simulink model "DataPath"  (R2025a)
settings: Solver=FixedStepAuto  StartTime=0  StopTime=0.02  FixedStep=1e-7  RelTol=1e-3
undefined symbols (not defined in the file): Bit_1, Bit_2, Bit_3, Bit_4, Bit_5, Bit_6, Bit_7, Bit_8
libraries: simulink_extras x126, fl_lib x34, nesl_utility x18, simulink x2
(part 7 of 7)

== system DataPath/Subsystem1/ALU Regs/B2/Subsystem4 ==
  Data : Inport
  Store : Inport  Port=2
  Clock : Inport  Port=3
  Clear : Inport  Port=4
  AND : Logic  IconShape=distinctive  AllPortsSameDT=off  OutDataTypeStr=boolean
  AND1 : Logic  IconShape=distinctive  AllPortsSameDT=off  OutDataTypeStr=boolean
  D Flip-Flop : simulink_extras/Flip Flops/D Flip-Flop
  NOT : Logic  Operator=NOT  IconShape=distinctive  AllPortsSameDT=off  OutDataTypeStr=boolean
  NOT1 : Logic  Operator=NOT  IconShape=distinctive  AllPortsSameDT=off  OutDataTypeStr=boolean
  OR : Logic  Operator=OR  IconShape=distinctive  AllPortsSameDT=off  OutDataTypeStr=boolean
  Q : Outport
  !Q : Outport  Port=2
  wires:
  AND1/1 -> OR/2
  AND/1 -> OR/1
  D Flip-Flop/1 -> Q/1, AND1/2
  NOT/1 -> AND1/1
  Store/1 -> AND/2, NOT/1
  Clock/1 -> D Flip-Flop/2
  Data/1 -> AND/1
  OR/1 -> D Flip-Flop/1
  D Flip-Flop/2 -> !Q/1
  Clear/1 -> NOT1/1
  NOT1/1 -> D Flip-Flop/3

== system DataPath/Subsystem1/ALU Regs/B2/Subsystem5 ==
  Data : Inport
  Store : Inport  Port=2
  Clock : Inport  Port=3
  Clear : Inport  Port=4
  AND : Logic  IconShape=distinctive  AllPortsSameDT=off  OutDataTypeStr=boolean
  AND1 : Logic  IconShape=distinctive  AllPortsSameDT=off  OutDataTypeStr=boolean
  D Flip-Flop : simulink_extras/Flip Flops/D Flip-Flop
  NOT : Logic  Operator=NOT  IconShape=distinctive  AllPortsSameDT=off  OutDataTypeStr=boolean
  NOT1 : Logic  Operator=NOT  IconShape=distinctive  AllPortsSameDT=off  OutDataTypeStr=boolean
  OR : Logic  Operator=OR  IconShape=distinctive  AllPortsSameDT=off  OutDataTypeStr=boolean
  Q : Outport
  !Q : Outport  Port=2
  wires:
  AND1/1 -> OR/2
  AND/1 -> OR/1
  D Flip-Flop/1 -> Q/1, AND1/2
  NOT/1 -> AND1/1
  Store/1 -> AND/2, NOT/1
  Clock/1 -> D Flip-Flop/2
  Data/1 -> AND/1
  OR/1 -> D Flip-Flop/1
  D Flip-Flop/2 -> !Q/1
  Clear/1 -> NOT1/1
  NOT1/1 -> D Flip-Flop/3

== system DataPath/Subsystem1/ALU Regs/B2/Subsystem6 ==
  Data : Inport
  Store : Inport  Port=2
  Clock : Inport  Port=3
  Clear : Inport  Port=4
  AND : Logic  IconShape=distinctive  AllPortsSameDT=off  OutDataTypeStr=boolean
  AND1 : Logic  IconShape=distinctive  AllPortsSameDT=off  OutDataTypeStr=boolean
  D Flip-Flop : simulink_extras/Flip Flops/D Flip-Flop
  NOT : Logic  Operator=NOT  IconShape=distinctive  AllPortsSameDT=off  OutDataTypeStr=boolean
  NOT1 : Logic  Operator=NOT  IconShape=distinctive  AllPortsSameDT=off  OutDataTypeStr=boolean
  OR : Logic  Operator=OR  IconShape=distinctive  AllPortsSameDT=off  OutDataTypeStr=boolean
  Q : Outport
  !Q : Outport  Port=2
  wires:
  AND1/1 -> OR/2
  AND/1 -> OR/1
  D Flip-Flop/1 -> Q/1, AND1/2
  NOT/1 -> AND1/1
  Store/1 -> AND/2, NOT/1
  Clock/1 -> D Flip-Flop/2
  Data/1 -> AND/1
  OR/1 -> D Flip-Flop/1
  D Flip-Flop/2 -> !Q/1
  Clear/1 -> NOT1/1
  NOT1/1 -> D Flip-Flop/3

== system DataPath/Subsystem1/ALU Regs/B2/Subsystem7 ==
  Data : Inport
  Store : Inport  Port=2
  Clock : Inport  Port=3
  Clear : Inport  Port=4
  AND : Logic  IconShape=distinctive  AllPortsSameDT=off  OutDataTypeStr=boolean
  AND1 : Logic  IconShape=distinctive  AllPortsSameDT=off  OutDataTypeStr=boolean
  D Flip-Flop : simulink_extras/Flip Flops/D Flip-Flop
  NOT : Logic  Operator=NOT  IconShape=distinctive  AllPortsSameDT=off  OutDataTypeStr=boolean
  NOT1 : Logic  Operator=NOT  IconShape=distinctive  AllPortsSameDT=off  OutDataTypeStr=boolean
  OR : Logic  Operator=OR  IconShape=distinctive  AllPortsSameDT=off  OutDataTypeStr=boolean
  Q : Outport
  !Q : Outport  Port=2
  wires:
  AND1/1 -> OR/2
  AND/1 -> OR/1
  D Flip-Flop/1 -> Q/1, AND1/2
  NOT/1 -> AND1/1
  Store/1 -> AND/2, NOT/1
  Clock/1 -> D Flip-Flop/2
  Data/1 -> AND/1
  OR/1 -> D Flip-Flop/1
  D Flip-Flop/2 -> !Q/1
  Clear/1 -> NOT1/1
  NOT1/1 -> D Flip-Flop/3

== system DataPath/Subsystem1/ALU Regs/B2/Subsystem8 ==
  Data : Inport
  Store : Inport  Port=2
  Clock : Inport  Port=3
  Clear : Inport  Port=4
  AND : Logic  IconShape=distinctive  AllPortsSameDT=off  OutDataTypeStr=boolean
  AND1 : Logic  IconShape=distinctive  AllPortsSameDT=off  OutDataTypeStr=boolean
  D Flip-Flop : simulink_extras/Flip Flops/D Flip-Flop
  NOT : Logic  Operator=NOT  IconShape=distinctive  AllPortsSameDT=off  OutDataTypeStr=boolean
  NOT1 : Logic  Operator=NOT  IconShape=distinctive  AllPortsSameDT=off  OutDataTypeStr=boolean
  OR : Logic  Operator=OR  IconShape=distinctive  AllPortsSameDT=off  OutDataTypeStr=boolean
  Q : Outport
  !Q : Outport  Port=2
  wires:
  AND1/1 -> OR/2
  AND/1 -> OR/1
  D Flip-Flop/1 -> Q/1, AND1/2
  NOT/1 -> AND1/1
  Store/1 -> AND/2, NOT/1
  Clock/1 -> D Flip-Flop/2
  Data/1 -> AND/1
  OR/1 -> D Flip-Flop/1
  D Flip-Flop/2 -> !Q/1
  Clear/1 -> NOT1/1
  NOT1/1 -> D Flip-Flop/3

== system DataPath/Subsystem1/Normalize Div/Subsystem1/Subsystem6 ==
  Data : Inport
  CLK : Inport  Port=2
  Delay One Step : Delay  DelayLength=1
  NAND{1..4} (4 alike) : Logic  Operator=NAND  IconShape=distinctive  AllPortsSameDT=off  OutDataTypeStr=boolean
  Q : Outport
  !Q : Outport  Port=2
  wires:
  NAND1/1 -> Delay One Step/1
  NAND4/1 -> NAND2/2
  Delay One Step/1 -> NAND2/1, Q/1  "Q"
  NAND2/1 -> !Q/1, NAND1/2
  NAND3/1 -> NAND4/1, NAND1/1
  CLK/1 -> NAND3/2, NAND4/2
  Data/1 -> NAND3/1

== system DataPath/Subsystem1/Normalize Div/Subsystem1/Subsystem7 ==
  Data : Inport
  CLK : Inport  Port=2
  Delay One Step : Delay  DelayLength=1
  NAND{1..4} (4 alike) : Logic  Operator=NAND  IconShape=distinctive  AllPortsSameDT=off  OutDataTypeStr=boolean
  Q : Outport
  !Q : Outport  Port=2
  wires:
  NAND1/1 -> Delay One Step/1
  NAND4/1 -> NAND2/2
  Delay One Step/1 -> NAND2/1, Q/1  "Q"
  NAND2/1 -> !Q/1, NAND1/2
  NAND3/1 -> NAND4/1, NAND1/1
  CLK/1 -> NAND3/2, NAND4/2
  Data/1 -> NAND3/1

== system DataPath/Subsystem1/Normalize Div/Subsystem8/Subsystem6 ==
  Data : Inport
  CLK : Inport  Port=2
  Delay One Step : Delay  DelayLength=1
  NAND{1..4} (4 alike) : Logic  Operator=NAND  IconShape=distinctive  AllPortsSameDT=off  OutDataTypeStr=boolean
  Q : Outport
  !Q : Outport  Port=2
  wires:
  NAND1/1 -> Delay One Step/1
  NAND4/1 -> NAND2/2
  Delay One Step/1 -> NAND2/1, Q/1  "Q"
  NAND2/1 -> !Q/1, NAND1/2
  NAND3/1 -> NAND4/1, NAND1/1
  CLK/1 -> NAND3/2, NAND4/2
  Data/1 -> NAND3/1

== system DataPath/Subsystem1/Normalize Div/Subsystem8/Subsystem7 ==
  Data : Inport
  CLK : Inport  Port=2
  Delay One Step : Delay  DelayLength=1
  NAND{1..4} (4 alike) : Logic  Operator=NAND  IconShape=distinctive  AllPortsSameDT=off  OutDataTypeStr=boolean
  Q : Outport
  !Q : Outport  Port=2
  wires:
  NAND1/1 -> Delay One Step/1
  NAND4/1 -> NAND2/2
  Delay One Step/1 -> NAND2/1, Q/1  "Q"
  NAND2/1 -> !Q/1, NAND1/2
  NAND3/1 -> NAND4/1, NAND1/1
  CLK/1 -> NAND3/2, NAND4/2
  Data/1 -> NAND3/1

== system DataPath/Subsystem1/Stepper/Subsystem1/DFF ==
  Data : Inport
  CLK : Inport  Port=2
  DLatch Master : Subsystem
  DLatch Slave : Subsystem
  NOT6 : Logic  Operator=NOT  IconShape=distinctive  AllPortsSameDT=off  OutDataTypeStr=boolean
  Q : Outport
  !Q : Outport  Port=2
  wires:
  DLatch Master/1(Q) -> DLatch Slave/1(Data)
  NOT6/1 -> DLatch Master/2(CLK)
  CLK/1 -> DLatch Slave/2(CLK), NOT6/1
  Data/1 -> DLatch Master/1(Data)
  DLatch Slave/1(Q) -> Q/1
  DLatch Slave/2(!Q) -> !Q/1

== system DataPath/Subsystem1/Stepper/Subsystem2/DFF ==
  Data : Inport
  CLK : Inport  Port=2
  DLatch Master : Subsystem
  DLatch Slave : Subsystem
  NOT6 : Logic  Operator=NOT  IconShape=distinctive  AllPortsSameDT=off  OutDataTypeStr=boolean
  Q : Outport
  !Q : Outport  Port=2
  wires:
  DLatch Master/1(Q) -> DLatch Slave/1(Data)
  NOT6/1 -> DLatch Master/2(CLK)
  CLK/1 -> DLatch Slave/2(CLK), NOT6/1
  Data/1 -> DLatch Master/1(Data)
  DLatch Slave/1(Q) -> Q/1
  DLatch Slave/2(!Q) -> !Q/1

== system DataPath/Subsystem1/Stepper/Subsystem3/DFF ==
  Data : Inport
  CLK : Inport  Port=2
  DLatch Master : Subsystem
  DLatch Slave : Subsystem
  NOT6 : Logic  Operator=NOT  IconShape=distinctive  AllPortsSameDT=off  OutDataTypeStr=boolean
  Q : Outport
  !Q : Outport  Port=2
  wires:
  DLatch Master/1(Q) -> DLatch Slave/1(Data)
  NOT6/1 -> DLatch Master/2(CLK)
  CLK/1 -> DLatch Slave/2(CLK), NOT6/1
  Data/1 -> DLatch Master/1(Data)
  DLatch Slave/1(Q) -> Q/1
  DLatch Slave/2(!Q) -> !Q/1

== system DataPath/Subsystem1/Stepper/Subsystem4/DFF ==
  Data : Inport
  CLK : Inport  Port=2
  DLatch Master : Subsystem
  DLatch Slave : Subsystem
  NOT6 : Logic  Operator=NOT  IconShape=distinctive  AllPortsSameDT=off  OutDataTypeStr=boolean
  Q : Outport
  !Q : Outport  Port=2
  wires:
  DLatch Master/1(Q) -> DLatch Slave/1(Data)
  NOT6/1 -> DLatch Master/2(CLK)
  CLK/1 -> DLatch Slave/2(CLK), NOT6/1
  Data/1 -> DLatch Master/1(Data)
  DLatch Slave/1(Q) -> Q/1
  DLatch Slave/2(!Q) -> !Q/1

== system DataPath/Subsystem/Stepper/Subsystem1/DFF/DLatch Master ==
  Data : Inport
  CLK : Inport  Port=2
  Delay One Step : Delay  DelayLength=1
  NAND{1..4} (4 alike) : Logic  Operator=NAND  IconShape=distinctive  AllPortsSameDT=off  OutDataTypeStr=boolean
  Q : Outport
  !Q : Outport  Port=2
  wires:
  NAND1/1 -> Delay One Step/1
  NAND4/1 -> NAND2/2
  Delay One Step/1 -> NAND2/1, Q/1  "Q"
  NAND2/1 -> !Q/1, NAND1/2
  NAND3/1 -> NAND4/1, NAND1/1
  CLK/1 -> NAND3/2, NAND4/2
  Data/1 -> NAND3/1

== system DataPath/Subsystem/Stepper/Subsystem1/DFF/DLatch Slave ==
  Data : Inport
  CLK : Inport  Port=2
  Delay One Step : Delay  DelayLength=1
  NAND{1..4} (4 alike) : Logic  Operator=NAND  IconShape=distinctive  AllPortsSameDT=off  OutDataTypeStr=boolean
  Q : Outport
  !Q : Outport  Port=2
  wires:
  NAND1/1 -> Delay One Step/1
  NAND4/1 -> NAND2/2
  Delay One Step/1 -> NAND2/1, Q/1  "Q"
  NAND2/1 -> !Q/1, NAND1/2
  NAND3/1 -> NAND4/1, NAND1/1
  CLK/1 -> NAND3/2, NAND4/2
  Data/1 -> NAND3/1

== system DataPath/Subsystem/Stepper/Subsystem2/DFF/DLatch Master ==
  Data : Inport
  CLK : Inport  Port=2
  Delay One Step : Delay  DelayLength=1
  NAND{1..4} (4 alike) : Logic  Operator=NAND  IconShape=distinctive  AllPortsSameDT=off  OutDataTypeStr=boolean
  Q : Outport
  !Q : Outport  Port=2
  wires:
  NAND1/1 -> Delay One Step/1
  NAND4/1 -> NAND2/2
  Delay One Step/1 -> NAND2/1, Q/1  "Q"
  NAND2/1 -> !Q/1, NAND1/2
  NAND3/1 -> NAND4/1, NAND1/1
  CLK/1 -> NAND3/2, NAND4/2
  Data/1 -> NAND3/1

== system DataPath/Subsystem/Stepper/Subsystem2/DFF/DLatch Slave ==
  Data : Inport
  CLK : Inport  Port=2
  Delay One Step : Delay  DelayLength=1
  NAND{1..4} (4 alike) : Logic  Operator=NAND  IconShape=distinctive  AllPortsSameDT=off  OutDataTypeStr=boolean
  Q : Outport
  !Q : Outport  Port=2
  wires:
  NAND1/1 -> Delay One Step/1
  NAND4/1 -> NAND2/2
  Delay One Step/1 -> NAND2/1, Q/1  "Q"
  NAND2/1 -> !Q/1, NAND1/2
  NAND3/1 -> NAND4/1, NAND1/1
  CLK/1 -> NAND3/2, NAND4/2
  Data/1 -> NAND3/1

== system DataPath/Subsystem/Stepper/Subsystem3/DFF/DLatch Master ==
  Data : Inport
  CLK : Inport  Port=2
  Delay One Step : Delay  DelayLength=1
  NAND{1..4} (4 alike) : Logic  Operator=NAND  IconShape=distinctive  AllPortsSameDT=off  OutDataTypeStr=boolean
  Q : Outport
  !Q : Outport  Port=2
  wires:
  NAND1/1 -> Delay One Step/1
  NAND4/1 -> NAND2/2
  Delay One Step/1 -> NAND2/1, Q/1  "Q"
  NAND2/1 -> !Q/1, NAND1/2
  NAND3/1 -> NAND4/1, NAND1/1
  CLK/1 -> NAND3/2, NAND4/2
  Data/1 -> NAND3/1

== system DataPath/Subsystem/Stepper/Subsystem3/DFF/DLatch Slave ==
  Data : Inport
  CLK : Inport  Port=2
  Delay One Step : Delay  DelayLength=1
  NAND{1..4} (4 alike) : Logic  Operator=NAND  IconShape=distinctive  AllPortsSameDT=off  OutDataTypeStr=boolean
  Q : Outport
  !Q : Outport  Port=2
  wires:
  NAND1/1 -> Delay One Step/1
  NAND4/1 -> NAND2/2
  Delay One Step/1 -> NAND2/1, Q/1  "Q"
  NAND2/1 -> !Q/1, NAND1/2
  NAND3/1 -> NAND4/1, NAND1/1
  CLK/1 -> NAND3/2, NAND4/2
  Data/1 -> NAND3/1

== system DataPath/Subsystem/Stepper/Subsystem4/DFF/DLatch Master ==
  Data : Inport
  CLK : Inport  Port=2
  Delay One Step : Delay  DelayLength=1
  NAND{1..4} (4 alike) : Logic  Operator=NAND  IconShape=distinctive  AllPortsSameDT=off  OutDataTypeStr=boolean
  Q : Outport
  !Q : Outport  Port=2
  wires:
  NAND1/1 -> Delay One Step/1
  NAND4/1 -> NAND2/2
  Delay One Step/1 -> NAND2/1, Q/1  "Q"
  NAND2/1 -> !Q/1, NAND1/2
  NAND3/1 -> NAND4/1, NAND1/1
  CLK/1 -> NAND3/2, NAND4/2
  Data/1 -> NAND3/1

== system DataPath/Subsystem/Stepper/Subsystem4/DFF/DLatch Slave ==
  Data : Inport
  CLK : Inport  Port=2
  Delay One Step : Delay  DelayLength=1
  NAND{1..4} (4 alike) : Logic  Operator=NAND  IconShape=distinctive  AllPortsSameDT=off  OutDataTypeStr=boolean
  Q : Outport
  !Q : Outport  Port=2
  wires:
  NAND1/1 -> Delay One Step/1
  NAND4/1 -> NAND2/2
  Delay One Step/1 -> NAND2/1, Q/1  "Q"
  NAND2/1 -> !Q/1, NAND1/2
  NAND3/1 -> NAND4/1, NAND1/1
  CLK/1 -> NAND3/2, NAND4/2
  Data/1 -> NAND3/1

== system DataPath/Subsystem1/Stepper/Subsystem1/DFF/DLatch Master ==
  Data : Inport
  CLK : Inport  Port=2
  Delay One Step : Delay  DelayLength=1
  NAND{1..4} (4 alike) : Logic  Operator=NAND  IconShape=distinctive  AllPortsSameDT=off  OutDataTypeStr=boolean
  Q : Outport
  !Q : Outport  Port=2
  wires:
  NAND1/1 -> Delay One Step/1
  NAND4/1 -> NAND2/2
  Delay One Step/1 -> NAND2/1, Q/1  "Q"
  NAND2/1 -> !Q/1, NAND1/2
  NAND3/1 -> NAND4/1, NAND1/1
  CLK/1 -> NAND3/2, NAND4/2
  Data/1 -> NAND3/1

== system DataPath/Subsystem1/Stepper/Subsystem1/DFF/DLatch Slave ==
  Data : Inport
  CLK : Inport  Port=2
  Delay One Step : Delay  DelayLength=1
  NAND{1..4} (4 alike) : Logic  Operator=NAND  IconShape=distinctive  AllPortsSameDT=off  OutDataTypeStr=boolean
  Q : Outport
  !Q : Outport  Port=2
  wires:
  NAND1/1 -> Delay One Step/1
  NAND4/1 -> NAND2/2
  Delay One Step/1 -> NAND2/1, Q/1  "Q"
  NAND2/1 -> !Q/1, NAND1/2
  NAND3/1 -> NAND4/1, NAND1/1
  CLK/1 -> NAND3/2, NAND4/2
  Data/1 -> NAND3/1

== system DataPath/Subsystem1/Stepper/Subsystem2/DFF/DLatch Master ==
  Data : Inport
  CLK : Inport  Port=2
  Delay One Step : Delay  DelayLength=1
  NAND{1..4} (4 alike) : Logic  Operator=NAND  IconShape=distinctive  AllPortsSameDT=off  OutDataTypeStr=boolean
  Q : Outport
  !Q : Outport  Port=2
  wires:
  NAND1/1 -> Delay One Step/1
  NAND4/1 -> NAND2/2
  Delay One Step/1 -> NAND2/1, Q/1  "Q"
  NAND2/1 -> !Q/1, NAND1/2
  NAND3/1 -> NAND4/1, NAND1/1
  CLK/1 -> NAND3/2, NAND4/2
  Data/1 -> NAND3/1

== system DataPath/Subsystem1/Stepper/Subsystem2/DFF/DLatch Slave ==
  Data : Inport
  CLK : Inport  Port=2
  Delay One Step : Delay  DelayLength=1
  NAND{1..4} (4 alike) : Logic  Operator=NAND  IconShape=distinctive  AllPortsSameDT=off  OutDataTypeStr=boolean
  Q : Outport
  !Q : Outport  Port=2
  wires:
  NAND1/1 -> Delay One Step/1
  NAND4/1 -> NAND2/2
  Delay One Step/1 -> NAND2/1, Q/1  "Q"
  NAND2/1 -> !Q/1, NAND1/2
  NAND3/1 -> NAND4/1, NAND1/1
  CLK/1 -> NAND3/2, NAND4/2
  Data/1 -> NAND3/1

== system DataPath/Subsystem1/Stepper/Subsystem3/DFF/DLatch Master ==
  Data : Inport
  CLK : Inport  Port=2
  Delay One Step : Delay  DelayLength=1
  NAND{1..4} (4 alike) : Logic  Operator=NAND  IconShape=distinctive  AllPortsSameDT=off  OutDataTypeStr=boolean
  Q : Outport
  !Q : Outport  Port=2
  wires:
  NAND1/1 -> Delay One Step/1
  NAND4/1 -> NAND2/2
  Delay One Step/1 -> NAND2/1, Q/1  "Q"
  NAND2/1 -> !Q/1, NAND1/2
  NAND3/1 -> NAND4/1, NAND1/1
  CLK/1 -> NAND3/2, NAND4/2
  Data/1 -> NAND3/1

== system DataPath/Subsystem1/Stepper/Subsystem3/DFF/DLatch Slave ==
  Data : Inport
  CLK : Inport  Port=2
  Delay One Step : Delay  DelayLength=1
  NAND{1..4} (4 alike) : Logic  Operator=NAND  IconShape=distinctive  AllPortsSameDT=off  OutDataTypeStr=boolean
  Q : Outport
  !Q : Outport  Port=2
  wires:
  NAND1/1 -> Delay One Step/1
  NAND4/1 -> NAND2/2
  Delay One Step/1 -> NAND2/1, Q/1  "Q"
  NAND2/1 -> !Q/1, NAND1/2
  NAND3/1 -> NAND4/1, NAND1/1
  CLK/1 -> NAND3/2, NAND4/2
  Data/1 -> NAND3/1

== system DataPath/Subsystem1/Stepper/Subsystem4/DFF/DLatch Master ==
  Data : Inport
  CLK : Inport  Port=2
  Delay One Step : Delay  DelayLength=1
  NAND{1..4} (4 alike) : Logic  Operator=NAND  IconShape=distinctive  AllPortsSameDT=off  OutDataTypeStr=boolean
  Q : Outport
  !Q : Outport  Port=2
  wires:
  NAND1/1 -> Delay One Step/1
  NAND4/1 -> NAND2/2
  Delay One Step/1 -> NAND2/1, Q/1  "Q"
  NAND2/1 -> !Q/1, NAND1/2
  NAND3/1 -> NAND4/1, NAND1/1
  CLK/1 -> NAND3/2, NAND4/2
  Data/1 -> NAND3/1

== system DataPath/Subsystem1/Stepper/Subsystem4/DFF/DLatch Slave ==
  Data : Inport
  CLK : Inport  Port=2
  Delay One Step : Delay  DelayLength=1
  NAND{1..4} (4 alike) : Logic  Operator=NAND  IconShape=distinctive  AllPortsSameDT=off  OutDataTypeStr=boolean
  Q : Outport
  !Q : Outport  Port=2
  wires:
  NAND1/1 -> Delay One Step/1
  NAND4/1 -> NAND2/2
  Delay One Step/1 -> NAND2/1, Q/1  "Q"
  NAND2/1 -> !Q/1, NAND1/2
  NAND3/1 -> NAND4/1, NAND1/1
  CLK/1 -> NAND3/2, NAND4/2
  Data/1 -> NAND3/1

== matlab function DataPath/Subsystem1/ALU Regs/MATLAB Function2 ==
  data: Binary input; Decimal output
function Decimal = fcn(Binary)
    % Ensure the input is an 8-bit signal
    assert(length(Binary) == 8, 'Input must be an 8-bit binary signal');
    % Convert the logical array (true/false) to a double array (1/0)
    Binary = double(Binary);
    % Calculate the decimal value
    Decimal = 0;
    for i = 1:8
        Decimal = Decimal + Binary(i) * 2^(8 - i);
    end
end

== matlab function DataPath/Subsystem1/ALU Regs/MATLAB Function3 ==
  data: Binary input; Decimal output
function Decimal = fcn(Binary)
    % Ensure the input is an 8-bit signal
    assert(length(Binary) == 8, 'Input must be an 8-bit binary signal');
    % Convert the logical array (true/false) to a double array (1/0)
    Binary = double(Binary);
    % Calculate the decimal value
    Decimal = 0;
    for i = 1:8
        Decimal = Decimal + Binary(i) * 2^(8 - i);
    end
end

== matlab function DataPath/Subsystem1/ALU Regs/Subsystem2/MATLAB Function ==
  data: A1 input; Select output; A2 input
function Select = TSB(A1, A2)
    if A1 == 1
        Select = 0;
    elseif A2 == 1
        Select = 1;
    elseif A1 == A2     
        Select = -1;
    else
        Select = -1; % This handles cases where A1 or A2 might be different than 0 or 1
    end
end

== matlab function DataPath/Subsystem1/ALU Regs/Subsystem4/MATLAB Function ==
  data: A1 input; Select output; A2 input
function Select = TSB(A1, A2)
    if A1 == 1
        Select = 0;
    elseif A2 == 1
        Select = 1;
    elseif A1 == A2     
        Select = -1;
    else
        Select = -1; % This handles cases where A1 or A2 might be different than 0 or 1
    end
end

== matlab function DataPath/Subsystem1/ALU/ALU MUX/MATLAB Function1 ==
  data: InputBus input; output output; Selection input
function output =  Enabler(InputBus, Selection)
    % InputBus: A 6-bit bus representing [SUM, AND, OR, XOR, NOTA, NOTB]
    % Selection: An 8-bit bus where only one bit is active at a time
    % Output: A single bit based on the selected input or shift operation
    
    % Initialize the output as double
    output = 0.0;
    
    % Convert all inputs to double
    SUM_bus = double(InputBus(1));
    
    % Check which selection bit is active and assign the corresponding input
    if Selection(1) == 1
        output = double(InputBus(1)); % SUM
    elseif Selection(2) == 1
        output = double(InputBus(2)); % AND
    elseif Selection(3) == 1
        output = double(InputBus(3)); % OR
    elseif Selection(4) == 1
        output = double(InputBus(4)); % XOR
    elseif Selection(5) == 1
        output = double(InputBus(5)); % NOTA
    elseif Selection(6) == 1
        output = double(InputBus(6)); % NOTB
    elseif Selection(7) == 1
        % Shift right operation on SUM bus
        output = double(bitshift(SUM_bus, -1));
    elseif Selection(8) == 1
        % Shift left operation on SUM bus
        output = double(bitshift(SUM_bus, 1));
    else
        % Default case
        output = 0.0;
    end
end

== matlab function DataPath/Subsystem1/Subsystem4/MATLAB Function ==
  data: MainInput input; Select output; ALU input
function Select = TSB(MainInput, ALU)
    if MainInput == 1
        Select = 0;
    elseif ALU == 1
        Select = 1;    
    elseif MainInput == ALU    
        Select = -1;
    else
        Select = -1; 
    end
end

== matlab function DataPath/Subsystem/ALU Regs/MATLAB Function ==
  data: Binary input; Decimal output
function Decimal = fcn(Binary)
    % Ensure the input is an 8-bit signal
    assert(length(Binary) == 8, 'Input must be an 8-bit binary signal');
    % Convert the logical array (true/false) to a double array (1/0)
    Binary = double(Binary);
    % Calculate the decimal value
    Decimal = 0;
    for i = 1:8
        Decimal = Decimal + Binary(i) * 2^(8 - i);
    end
end

== matlab function DataPath/Subsystem/ALU Regs/MATLAB Function1 ==
  data: Binary input; Decimal output
function Decimal = fcn(Binary)
    % Ensure the input is an 8-bit signal
    assert(length(Binary) == 8, 'Input must be an 8-bit binary signal');
    % Convert the logical array (true/false) to a double array (1/0)
    Binary = double(Binary);
    % Calculate the decimal value
    Decimal = 0;
    for i = 1:8
        Decimal = Decimal + Binary(i) * 2^(8 - i);
    end
end

== matlab function DataPath/Subsystem/ALU Regs/MATLAB Function2 ==
  data: Binary input; Decimal output
function Decimal = fcn(Binary)
    % Ensure the input is an 8-bit signal
    assert(length(Binary) == 8, 'Input must be an 8-bit binary signal');
    % Convert the logical array (true/false) to a double array (1/0)
    Binary = double(Binary);
    % Calculate the decimal value
    Decimal = 0;
    for i = 1:8
        Decimal = Decimal + Binary(i) * 2^(8 - i);
    end
end

== matlab function DataPath/Subsystem/ALU Regs/MATLAB Function3 ==
  data: Binary input; Decimal output
function Decimal = fcn(Binary)
    % Ensure the input is an 8-bit signal
    assert(length(Binary) == 8, 'Input must be an 8-bit binary signal');
    % Convert the logical array (true/false) to a double array (1/0)
    Binary = double(Binary);
    % Calculate the decimal value
    Decimal = 0;
    for i = 1:8
        Decimal = Decimal + Binary(i) * 2^(8 - i);
    end
end

== matlab function DataPath/Subsystem/ALU Regs/Subsystem2/MATLAB Function ==
  data: A1 input; Select output; A2 input
function Select = TSB(A1, A2)
    if A1 == 1
        Select = 0;
    elseif A2 == 1
        Select = 1;
    elseif A1 == A2     
        Select = -1;
    else
        Select = -1; % This handles cases where A1 or A2 might be different than 0 or 1
    end
end

== matlab function DataPath/Subsystem/ALU Regs/Subsystem4/MATLAB Function ==
  data: A1 input; Select output; A2 input
function Select = TSB(A1, A2)
    if A1 == 1
        Select = 0;
    elseif A2 == 1
        Select = 1;
    elseif A1 == A2     
        Select = -1;
    else
        Select = -1; % This handles cases where A1 or A2 might be different than 0 or 1
    end
end

== matlab function DataPath/Subsystem/ALU/ALU MUX/MATLAB Function1 ==
  data: InputBus input; output output; Selection input
function output =  Enabler(InputBus, Selection)
    % InputBus: A 6-bit bus representing [SUM, AND, OR, XOR, NOTA, NOTB]
    % Selection: An 8-bit bus where only one bit is active at a time
    % Output: A single bit based on the selected input or shift operation
    
    % Initialize the output as double
    output = 0.0;
    
    % Convert all inputs to double
    SUM_bus = double(InputBus(1));
    
    % Check which selection bit is active and assign the corresponding input
    if Selection(1) == 1
        output = double(InputBus(1)); % SUM
    elseif Selection(2) == 1
        output = double(InputBus(2)); % AND
    elseif Selection(3) == 1
        output = double(InputBus(3)); % OR
    elseif Selection(4) == 1
        output = double(InputBus(4)); % XOR
    elseif Selection(5) == 1
        output = double(InputBus(5)); % NOTA
    elseif Selection(6) == 1
        output = double(InputBus(6)); % NOTB
    elseif Selection(7) == 1
        % Shift right operation on SUM bus
        output = double(bitshift(SUM_bus, -1));
    elseif Selection(8) == 1
        % Shift left operation on SUM bus
        output = double(bitshift(SUM_bus, 1));
    else
        % Default case
        output = 0.0;
    end
end

== matlab function DataPath/Subsystem/ALU/ALU MUX/MATLAB Function2 ==
  data: InputBus input; output output; Selection input
function output =  Enabler(InputBus, Selection)
    % InputBus: A 6-bit bus representing [SUM, AND, OR, XOR, NOTA, NOTB]
    % Selection: An 8-bit bus where only one bit is active at a time
    % Output: A single bit based on the selected input or shift operation
    
    % Initialize the output as double
    output = 0.0;
    
    % Convert all inputs to double
    SUM_bus = double(InputBus(1));
    
    % Check which selection bit is active and assign the corresponding input
    if Selection(1) == 1
        output = double(InputBus(1)); % SUM
    elseif Selection(2) == 1
        output = double(InputBus(2)); % AND
    elseif Selection(3) == 1
        output = double(InputBus(3)); % OR
    elseif Selection(4) == 1
        output = double(InputBus(4)); % XOR
    elseif Selection(5) == 1
        output = double(InputBus(5)); % NOTA
    elseif Selection(6) == 1
        output = double(InputBus(6)); % NOTB
    elseif Selection(7) == 1
        % Shift right operation on SUM bus
        output = double(bitshift(SUM_bus, -1));
    elseif Selection(8) == 1
        % Shift left operation on SUM bus
        output = double(bitshift(SUM_bus, 1));
    else
        % Default case
        output = 0.0;
    end
end

== matlab function DataPath/Subsystem/ALU/ALU MUX/MATLAB Function3 ==
  data: InputBus input; output output; Selection input
function output =  Enabler(InputBus, Selection)
    % InputBus: A 6-bit bus representing [SUM, AND, OR, XOR, NOTA, NOTB]
    % Selection: An 8-bit bus where only one bit is active at a time
    % Output: A single bit based on the selected input or shift operation
    
    % Initialize the output as double
    output = 0.0;
    
    % Convert all inputs to double
    SUM_bus = double(InputBus(1));
    
    % Check which selection bit is active and assign the corresponding input
    if Selection(1) == 1
        output = double(InputBus(1)); % SUM
    elseif Selection(2) == 1
        output = double(InputBus(2)); % AND
    elseif Selection(3) == 1
        output = double(InputBus(3)); % OR
    elseif Selection(4) == 1
        output = double(InputBus(4)); % XOR
    elseif Selection(5) == 1
        output = double(InputBus(5)); % NOTA
    elseif Selection(6) == 1
        output = double(InputBus(6)); % NOTB
    elseif Selection(7) == 1
        % Shift right operation on SUM bus
        output = double(bitshift(SUM_bus, -1));
    elseif Selection(8) == 1
        % Shift left operation on SUM bus
        output = double(bitshift(SUM_bus, 1));
    else
        % Default case
        output = 0.0;
    end
end

== matlab function DataPath/Subsystem1/ALU/ALU MUX/MATLAB Function2 ==
  data: InputBus input; output output; Selection input
function output =  Enabler(InputBus, Selection)
    % InputBus: A 6-bit bus representing [SUM, AND, OR, XOR, NOTA, NOTB]
    % Selection: An 8-bit bus where only one bit is active at a time
    % Output: A single bit based on the selected input or shift operation
    
    % Initialize the output as double
    output = 0.0;
    
    % Convert all inputs to double
    SUM_bus = double(InputBus(1));
    
    % Check which selection bit is active and assign the corresponding input
    if Selection(1) == 1
        output = double(InputBus(1)); % SUM
    elseif Selection(2) == 1
        output = double(InputBus(2)); % AND
    elseif Selection(3) == 1
        output = double(InputBus(3)); % OR
    elseif Selection(4) == 1
        output = double(InputBus(4)); % XOR
    elseif Selection(5) == 1
        output = double(InputBus(5)); % NOTA
    elseif Selection(6) == 1
        output = double(InputBus(6)); % NOTB
    elseif Selection(7) == 1
        % Shift right operation on SUM bus
        output = double(bitshift(SUM_bus, -1));
    elseif Selection(8) == 1
        % Shift left operation on SUM bus
        output = double(bitshift(SUM_bus, 1));
    else
        % Default case
        output = 0.0;
    end
end

== matlab function DataPath/Subsystem/ALU/ALU MUX/MATLAB Function4 ==
  data: InputBus input; output output; Selection input
function output =  Enabler(InputBus, Selection)
    % InputBus: A 6-bit bus representing [SUM, AND, OR, XOR, NOTA, NOTB]
    % Selection: An 8-bit bus where only one bit is active at a time
    % Output: A single bit based on the selected input or shift operation
    
    % Initialize the output as double
    output = 0.0;
    
    % Convert all inputs to double
    SUM_bus = double(InputBus(1));
    
    % Check which selection bit is active and assign the corresponding input
    if Selection(1) == 1
        output = double(InputBus(1)); % SUM
    elseif Selection(2) == 1
        output = double(InputBus(2)); % AND
    elseif Selection(3) == 1
        output = double(InputBus(3)); % OR
    elseif Selection(4) == 1
        output = double(InputBus(4)); % XOR
    elseif Selection(5) == 1
        output = double(InputBus(5)); % NOTA
    elseif Selection(6) == 1
        output = double(InputBus(6)); % NOTB
    elseif Selection(7) == 1
        % Shift right operation on SUM bus
        output = double(bitshift(SUM_bus, -1));
    elseif Selection(8) == 1
        % Shift left operation on SUM bus
        output = double(bitshift(SUM_bus, 1));
    else
        % Default case
        output = 0.0;
    end
end

== matlab function DataPath/Subsystem/ALU/ALU MUX/MATLAB Function5 ==
  data: InputBus input; output output; Selection input
function output =  Enabler(InputBus, Selection)
    % InputBus: A 6-bit bus representing [SUM, AND, OR, XOR, NOTA, NOTB]
    % Selection: An 8-bit bus where only one bit is active at a time
    % Output: A single bit based on the selected input or shift operation
    
    % Initialize the output as double
    output = 0.0;
    
    % Convert all inputs to double
    SUM_bus = double(InputBus(1));
    
    % Check which selection bit is active and assign the corresponding input
    if Selection(1) == 1
        output = double(InputBus(1)); % SUM
    elseif Selection(2) == 1
        output = double(InputBus(2)); % AND
    elseif Selection(3) == 1
        output = double(InputBus(3)); % OR
    elseif Selection(4) == 1
        output = double(InputBus(4)); % XOR
    elseif Selection(5) == 1
        output = double(InputBus(5)); % NOTA
    elseif Selection(6) == 1
        output = double(InputBus(6)); % NOTB
    elseif Selection(7) == 1
        % Shift right operation on SUM bus
        output = double(bitshift(SUM_bus, -1));
    elseif Selection(8) == 1
        % Shift left operation on SUM bus
        output = double(bitshift(SUM_bus, 1));
    else
        % Default case
        output = 0.0;
    end
end

== matlab function DataPath/Subsystem/ALU/ALU MUX/MATLAB Function6 ==
  data: InputBus input; output output; Selection input
function output =  Enabler(InputBus, Selection)
    % InputBus: A 6-bit bus representing [SUM, AND, OR, XOR, NOTA, NOTB]
    % Selection: An 8-bit bus where only one bit is active at a time
    % Output: A single bit based on the selected input or shift operation
    
    % Initialize the output as double
    output = 0.0;
    
    % Convert all inputs to double
    SUM_bus = double(InputBus(1));
    
    % Check which selection bit is active and assign the corresponding input
    if Selection(1) == 1
        output = double(InputBus(1)); % SUM
    elseif Selection(2) == 1
        output = double(InputBus(2)); % AND
    elseif Selection(3) == 1
        output = double(InputBus(3)); % OR
    elseif Selection(4) == 1
        output = double(InputBus(4)); % XOR
    elseif Selection(5) == 1
        output = double(InputBus(5)); % NOTA
    elseif Selection(6) == 1
        output = double(InputBus(6)); % NOTB
    elseif Selection(7) == 1
        % Shift right operation on SUM bus
        output = double(bitshift(SUM_bus, -1));
    elseif Selection(8) == 1
        % Shift left operation on SUM bus
        output = double(bitshift(SUM_bus, 1));
    else
        % Default case
        output = 0.0;
    end
end

== matlab function DataPath/Subsystem/ALU/ALU MUX/MATLAB Function7 ==
  data: InputBus input; output output; Selection input
function output =  Enabler(InputBus, Selection)
    % InputBus: A 6-bit bus representing [SUM, AND, OR, XOR, NOTA, NOTB]
    % Selection: An 8-bit bus where only one bit is active at a time
    % Output: A single bit based on the selected input or shift operation
    
    % Initialize the output as double
    output = 0.0;
    
    % Convert all inputs to double
    SUM_bus = double(InputBus(1));
    
    % Check which selection bit is active and assign the corresponding input
    if Selection(1) == 1
        output = double(InputBus(1)); % SUM
    elseif Selection(2) == 1
        output = double(InputBus(2)); % AND
    elseif Selection(3) == 1
        output = double(InputBus(3)); % OR
    elseif Selection(4) == 1
        output = double(InputBus(4)); % XOR
    elseif Selection(5) == 1
        output = double(InputBus(5)); % NOTA
    elseif Selection(6) == 1
        output = double(InputBus(6)); % NOTB
    elseif Selection(7) == 1
        % Shift right operation on SUM bus
        output = double(bitshift(SUM_bus, -1));
    elseif Selection(8) == 1
        % Shift left operation on SUM bus
        output = double(bitshift(SUM_bus, 1));
    else
        % Default case
        output = 0.0;
    end
end

== matlab function DataPath/Subsystem/ALU/ALU MUX/MATLAB Function8 ==
  data: InputBus input; output output; Selection input
function output =  Enabler(InputBus, Selection)
    % InputBus: A 6-bit bus representing [SUM, AND, OR, XOR, NOTA, NOTB]
    % Selection: An 8-bit bus where only one bit is active at a time
    % Output: A single bit based on the selected input or shift operation
    
    % Initialize the output as double
    output = 0.0;
    
    % Convert all inputs to double
    SUM_bus = double(InputBus(1));
    
    % Check which selection bit is active and assign the corresponding input
    if Selection(1) == 1
        output = double(InputBus(1)); % SUM
    elseif Selection(2) == 1
        output = double(InputBus(2)); % AND
    elseif Selection(3) == 1
        output = double(InputBus(3)); % OR
    elseif Selection(4) == 1
        output = double(InputBus(4)); % XOR
    elseif Selection(5) == 1
        output = double(InputBus(5)); % NOTA
    elseif Selection(6) == 1
        output = double(InputBus(6)); % NOTB
    elseif Selection(7) == 1
        % Shift right operation on SUM bus
        output = double(bitshift(SUM_bus, -1));
    elseif Selection(8) == 1
        % Shift left operation on SUM bus
        output = double(bitshift(SUM_bus, 1));
    else
        % Default case
        output = 0.0;
    end
end

== matlab function DataPath/Subsystem/ALU/Adder & Logic Module/MATLAB Function1 ==
  data: Binary input; Decimal output
function Decimal = fcn(Binary)
    % Ensure the input is an 8-bit signal
    assert(length(Binary) == 8, 'Input must be an 8-bit binary signal');
    % Convert the logical array (true/false) to a double array (1/0)
    Binary = double(Binary);
    % Calculate the decimal value
    Decimal = 0;
    for i = 1:8
        Decimal = Decimal + Binary(i) * 2^(8 - i);
    end
end

== matlab function DataPath/Subsystem/ALU/Adder & Logic Module/MATLAB Function3 ==
  data: Binary input; Decimal output
function Decimal = fcn(Binary)
    % Ensure the input is an 8-bit signal
    assert(length(Binary) == 8, 'Input must be an 8-bit binary signal');
    % Convert the logical array (true/false) to a double array (1/0)
    Binary = double(Binary);
    % Calculate the decimal value
    Decimal = 0;
    for i = 1:8
        Decimal = Decimal + Binary(i) * 2^(8 - i);
    end
end

== matlab function DataPath/Subsystem/Subsystem4/MATLAB Function ==
  data: MainInput input; Select output; ALU input
function Select = TSB(MainInput, ALU)
    if MainInput == 1
        Select = 0;
    elseif ALU == 1
        Select = 1;    
    elseif MainInput == ALU    
        Select = -1;
    else
        Select = -1; 
    end
end

== matlab function DataPath/Subsystem1/ALU/ALU MUX/MATLAB Function3 ==
  data: InputBus input; output output; Selection input
function output =  Enabler(InputBus, Selection)
    % InputBus: A 6-bit bus representing [SUM, AND, OR, XOR, NOTA, NOTB]
    % Selection: An 8-bit bus where only one bit is active at a time
    % Output: A single bit based on the selected input or shift operation
    
    % Initialize the output as double
    output = 0.0;
    
    % Convert all inputs to double
    SUM_bus = double(InputBus(1));
    
    % Check which selection bit is active and assign the corresponding input
    if Selection(1) == 1
        output = double(InputBus(1)); % SUM
    elseif Selection(2) == 1
        output = double(InputBus(2)); % AND
    elseif Selection(3) == 1
        output = double(InputBus(3)); % OR
    elseif Selection(4) == 1
        output = double(InputBus(4)); % XOR
    elseif Selection(5) == 1
        output = double(InputBus(5)); % NOTA
    elseif Selection(6) == 1
        output = double(InputBus(6)); % NOTB
    elseif Selection(7) == 1
        % Shift right operation on SUM bus
        output = double(bitshift(SUM_bus, -1));
    elseif Selection(8) == 1
        % Shift left operation on SUM bus
        output = double(bitshift(SUM_bus, 1));
    else
        % Default case
        output = 0.0;
    end
end

== matlab function DataPath/Subsystem1/ALU/ALU MUX/MATLAB Function4 ==
  data: InputBus input; output output; Selection input
function output =  Enabler(InputBus, Selection)
    % InputBus: A 6-bit bus representing [SUM, AND, OR, XOR, NOTA, NOTB]
    % Selection: An 8-bit bus where only one bit is active at a time
    % Output: A single bit based on the selected input or shift operation
    
    % Initialize the output as double
    output = 0.0;
    
    % Convert all inputs to double
    SUM_bus = double(InputBus(1));
    
    % Check which selection bit is active and assign the corresponding input
    if Selection(1) == 1
        output = double(InputBus(1)); % SUM
    elseif Selection(2) == 1
        output = double(InputBus(2)); % AND
    elseif Selection(3) == 1
        output = double(InputBus(3)); % OR
    elseif Selection(4) == 1
        output = double(InputBus(4)); % XOR
    elseif Selection(5) == 1
        output = double(InputBus(5)); % NOTA
    elseif Selection(6) == 1
        output = double(InputBus(6)); % NOTB
    elseif Selection(7) == 1
        % Shift right operation on SUM bus
        output = double(bitshift(SUM_bus, -1));
    elseif Selection(8) == 1
        % Shift left operation on SUM bus
        output = double(bitshift(SUM_bus, 1));
    else
        % Default case
        output = 0.0;
    end
end

== matlab function DataPath/Subsystem1/ALU/ALU MUX/MATLAB Function5 ==
  data: InputBus input; output output; Selection input
function output =  Enabler(InputBus, Selection)
    % InputBus: A 6-bit bus representing [SUM, AND, OR, XOR, NOTA, NOTB]
    % Selection: An 8-bit bus where only one bit is active at a time
    % Output: A single bit based on the selected input or shift operation
    
    % Initialize the output as double
    output = 0.0;
    
    % Convert all inputs to double
    SUM_bus = double(InputBus(1));
    
    % Check which selection bit is active and assign the corresponding input
    if Selection(1) == 1
        output = double(InputBus(1)); % SUM
    elseif Selection(2) == 1
        output = double(InputBus(2)); % AND
    elseif Selection(3) == 1
        output = double(InputBus(3)); % OR
    elseif Selection(4) == 1
        output = double(InputBus(4)); % XOR
    elseif Selection(5) == 1
        output = double(InputBus(5)); % NOTA
    elseif Selection(6) == 1
        output = double(InputBus(6)); % NOTB
    elseif Selection(7) == 1
        % Shift right operation on SUM bus
        output = double(bitshift(SUM_bus, -1));
    elseif Selection(8) == 1
        % Shift left operation on SUM bus
        output = double(bitshift(SUM_bus, 1));
    else
        % Default case
        output = 0.0;
    end
end

== matlab function DataPath/Subsystem1/ALU/ALU MUX/MATLAB Function6 ==
  data: InputBus input; output output; Selection input
function output =  Enabler(InputBus, Selection)
    % InputBus: A 6-bit bus representing [SUM, AND, OR, XOR, NOTA, NOTB]
    % Selection: An 8-bit bus where only one bit is active at a time
    % Output: A single bit based on the selected input or shift operation
    
    % Initialize the output as double
    output = 0.0;
    
    % Convert all inputs to double
    SUM_bus = double(InputBus(1));
    
    % Check which selection bit is active and assign the corresponding input
    if Selection(1) == 1
        output = double(InputBus(1)); % SUM
    elseif Selection(2) == 1
        output = double(InputBus(2)); % AND
    elseif Selection(3) == 1
        output = double(InputBus(3)); % OR
    elseif Selection(4) == 1
        output = double(InputBus(4)); % XOR
    elseif Selection(5) == 1
        output = double(InputBus(5)); % NOTA
    elseif Selection(6) == 1
        output = double(InputBus(6)); % NOTB
    elseif Selection(7) == 1
        % Shift right operation on SUM bus
        output = double(bitshift(SUM_bus, -1));
    elseif Selection(8) == 1
        % Shift left operation on SUM bus
        output = double(bitshift(SUM_bus, 1));
    else
        % Default case
        output = 0.0;
    end
end

== matlab function DataPath/Subsystem1/ALU/ALU MUX/MATLAB Function7 ==
  data: InputBus input; output output; Selection input
function output =  Enabler(InputBus, Selection)
    % InputBus: A 6-bit bus representing [SUM, AND, OR, XOR, NOTA, NOTB]
    % Selection: An 8-bit bus where only one bit is active at a time
    % Output: A single bit based on the selected input or shift operation
    
    % Initialize the output as double
    output = 0.0;
    
    % Convert all inputs to double
    SUM_bus = double(InputBus(1));
    
    % Check which selection bit is active and assign the corresponding input
    if Selection(1) == 1
        output = double(InputBus(1)); % SUM
    elseif Selection(2) == 1
        output = double(InputBus(2)); % AND
    elseif Selection(3) == 1
        output = double(InputBus(3)); % OR
    elseif Selection(4) == 1
        output = double(InputBus(4)); % XOR
    elseif Selection(5) == 1
        output = double(InputBus(5)); % NOTA
    elseif Selection(6) == 1
        output = double(InputBus(6)); % NOTB
    elseif Selection(7) == 1
        % Shift right operation on SUM bus
        output = double(bitshift(SUM_bus, -1));
    elseif Selection(8) == 1
        % Shift left operation on SUM bus
        output = double(bitshift(SUM_bus, 1));
    else
        % Default case
        output = 0.0;
    end
end

== matlab function DataPath/Subsystem1/ALU/ALU MUX/MATLAB Function8 ==
  data: InputBus input; output output; Selection input
function output =  Enabler(InputBus, Selection)
    % InputBus: A 6-bit bus representing [SUM, AND, OR, XOR, NOTA, NOTB]
    % Selection: An 8-bit bus where only one bit is active at a time
    % Output: A single bit based on the selected input or shift operation
    
    % Initialize the output as double
    output = 0.0;
    
    % Convert all inputs to double
    SUM_bus = double(InputBus(1));
    
    % Check which selection bit is active and assign the corresponding input
    if Selection(1) == 1
        output = double(InputBus(1)); % SUM
    elseif Selection(2) == 1
        output = double(InputBus(2)); % AND
    elseif Selection(3) == 1
        output = double(InputBus(3)); % OR
    elseif Selection(4) == 1
        output = double(InputBus(4)); % XOR
    elseif Selection(5) == 1
        output = double(InputBus(5)); % NOTA
    elseif Selection(6) == 1
        output = double(InputBus(6)); % NOTB
    elseif Selection(7) == 1
        % Shift right operation on SUM bus
        output = double(bitshift(SUM_bus, -1));
    elseif Selection(8) == 1
        % Shift left operation on SUM bus
        output = double(bitshift(SUM_bus, 1));
    else
        % Default case
        output = 0.0;
    end
end

== matlab function DataPath/Subsystem1/ALU/Adder & Logic Module/MATLAB Function1 ==
  data: Binary input; Decimal output
function Decimal = fcn(Binary)
    % Ensure the input is an 8-bit signal
    assert(length(Binary) == 8, 'Input must be an 8-bit binary signal');
    % Convert the logical array (true/false) to a double array (1/0)
    Binary = double(Binary);
    % Calculate the decimal value
    Decimal = 0;
    for i = 1:8
        Decimal = Decimal + Binary(i) * 2^(8 - i);
    end
end

== matlab function DataPath/Subsystem1/ALU/Adder & Logic Module/MATLAB Function3 ==
  data: Binary input; Decimal output
function Decimal = fcn(Binary)
    % Ensure the input is an 8-bit signal
    assert(length(Binary) == 8, 'Input must be an 8-bit binary signal');
    % Convert the logical array (true/false) to a double array (1/0)
    Binary = double(Binary);
    % Calculate the decimal value
    Decimal = 0;
    for i = 1:8
        Decimal = Decimal + Binary(i) * 2^(8 - i);
    end
end

== matlab function DataPath/Subsystem1/ALU Regs/MATLAB Function ==
  data: Binary input; Decimal output
function Decimal = fcn(Binary)
    % Ensure the input is an 8-bit signal
    assert(length(Binary) == 8, 'Input must be an 8-bit binary signal');
    % Convert the logical array (true/false) to a double array (1/0)
    Binary = double(Binary);
    % Calculate the decimal value
    Decimal = 0;
    for i = 1:8
        Decimal = Decimal + Binary(i) * 2^(8 - i);
    end
end

== matlab function DataPath/Subsystem1/ALU Regs/MATLAB Function1 ==
  data: Binary input; Decimal output
function Decimal = fcn(Binary)
    % Ensure the input is an 8-bit signal
    assert(length(Binary) == 8, 'Input must be an 8-bit binary signal');
    % Convert the logical array (true/false) to a double array (1/0)
    Binary = double(Binary);
    % Calculate the decimal value
    Decimal = 0;
    for i = 1:8
        Decimal = Decimal + Binary(i) * 2^(8 - i);
    end
end
